simulink model "virtualOptim"  (R2013a)
settings: Solver=FixedStepDiscrete  StartTime=0.0  StopTime=10.0  RelTol=1e-3
settings Model: Creator=bbhattac  LastModifiedBy=bbhattac
settings OptimizationCC: InlineParams=on  ExpressionDepthLimit=2147483647  OptimizeModelRefInitCode=on  LifeSpan=1
settings DebuggingCC: ParameterPrecisionLossMsg=none  FcnCallInpInsideContextMsg=UseLocalSettings  StrictBusMsg=Warning
settings RTWCC: SystemTargetFile=ert.tlc  GenCodeOnly=on  TemplateMakefile=ert_default_tmf  Description=Real-Time Workshop Embedded Coder  GenerateReport=on  ProcessScript=ert_make_rtw_hook  IncludeHyperlinkInReport=on  LaunchReport=on  GenerateTraceInfo=on  GenerateTraceReport=on  GenerateTraceReportSl=on  GenerateTraceReportSf=on  GenerateTraceReportEml=on
settings CodeAppCC: IgnoreCustomStorageClasses=off  CustomSymbolStrType=$N$R$M  InternalIdentifier=Classic
settings ERTTargetCC: InlinedParameterPlacement=Hierarchical  ERTCustomFileTemplate=example_file_process.tlc

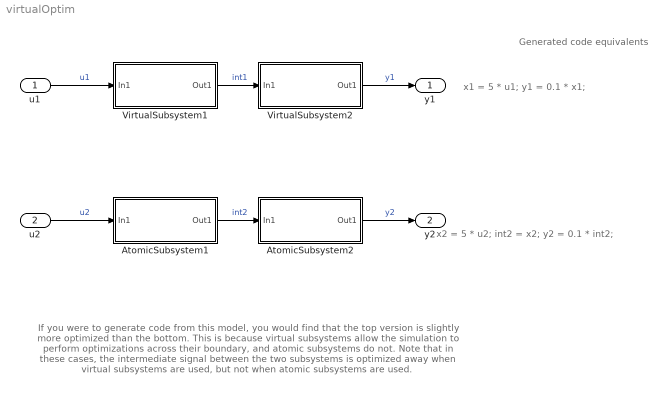
== system virtualOptim ==
  note: Generated code equivalents
  note: x2 = 5 * u2;
      | int2 = x2;
      | y2 = 0.1 * int2;
  note: x1 = 5 * u1;
      | y1 = 0.1 * x1;
  note: If you were to generate code from this model, you would
      | find that the top version is slightly more optimized than the
      | bottom.  This is because virtual subsystems allow the simulation
      | to perform optimizations across their boundary, and atomic
      | subsystems do not.  Note that in these cases, the intermediate
      | signal between the two subsystems is optimized away when
      | virtual subsystems are used, but not when atomic subsystems
      | are used.
  u1 : Inport  PortDimensions=1
  u2 : Inport  Port=2  PortDimensions=1
  AtomicSubsystem1 : Subsystem  TreatAsAtomicUnit=on
  AtomicSubsystem2 : Subsystem  TreatAsAtomicUnit=on
  VirtualSubsystem1 : Subsystem
  VirtualSubsystem2 : Subsystem
  y1 : Outport
  y2 : Outport  Port=2
  wires:
  VirtualSubsystem1/1(Out1) -> VirtualSubsystem2/1(In1)  "int1"
  VirtualSubsystem2/1(Out1) -> y1/1  "y1"
  u1/1 -> VirtualSubsystem1/1(In1)  "u1"
  AtomicSubsystem1/1(Out1) -> AtomicSubsystem2/1(In1)  "int2"
  AtomicSubsystem2/1(Out1) -> y2/1  "y2"
  u2/1 -> AtomicSubsystem1/1(In1)  "u2"

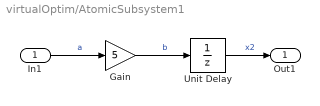
== system virtualOptim/AtomicSubsystem1 ==
  In1 : Inport
  Gain : Gain  Gain=5
  Unit Delay : UnitDelay  SampleTime=-1
  Out1 : Outport
  wires:
  Unit Delay/1 -> Out1/1  "x2"
  In1/1 -> Gain/1  "a"
  Gain/1 -> Unit Delay/1  "b"

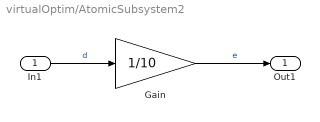
== system virtualOptim/AtomicSubsystem2 ==
  In1 : Inport
  Gain : Gain  Gain=1/10
  Out1 : Outport
  wires:
  Gain/1 -> Out1/1  "e"
  In1/1 -> Gain/1  "d"

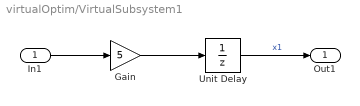
== system virtualOptim/VirtualSubsystem1 ==
  In1 : Inport
  Gain : Gain  Gain=5
  Unit Delay : UnitDelay  SampleTime=-1
  Out1 : Outport
  wires:
  Unit Delay/1 -> Out1/1  "x1"
  Gain/1 -> Unit Delay/1
  In1/1 -> Gain/1

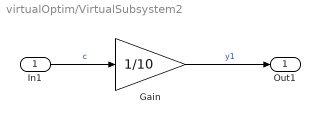
== system virtualOptim/VirtualSubsystem2 ==
  In1 : Inport
  Gain : Gain  Gain=1/10
  Out1 : Outport
  wires:
  In1/1 -> Gain/1  "c"
  Gain/1 -> Out1/1  "y1"
